simulink library "EmE_MBD_Blockset"  (R2018a)
settings: Solver=ode1  StartTime=0.0  StopTime=Inf  FixedStep=0.001  RelTol=1e-3  EnableMultiTasking=on
PostLoadFcn:
  | , if any(exist('dsrtsu_mdlpostloadfcn', 'file') == [2, 3, 6]), try dsrtsu_mdlpostloadfcn('Execute', bdroot); catch fprintf('Error in PostLoadFcn (dsrtsu_mdlpostloadfcn) for model "%s":\n %s\n', bdroot, lasterr); end, end,
undefined symbols (not defined in the file or in its folder): ENUM_TSC1_CONTROL_PURPOSE_T, gcbh, GLB_SWITCH_T
libraries: simulink x237, $bdroot x115, simulink_need_slupdate x26, MotoHawk_lib x13, simulink_extras x3
(part 8 of 11)

== system EmE_MBD_Blockset/User-Defined Functions/Snoop/CCP_ETC_SS1/Signal Data Pairing/Update Signal6/Reset Logic ==
  CurrentPID : Inport
  ResetDAQ : Inport  Port=2
  CCP_SNOOP_DAQSIZE : Constant  Value=16  OutDataTypeStr=uint8
  CCP_SNOOP_FIRSTPID : Constant  Value=64  OutDataTypeStr=uint8
  Divide : Product  Inputs=*/
  Logical Operator : Logic  Operator=OR  AllPortsSameDT=off  OutDataTypeStr=boolean
  Relational Operator : RelationalOperator  Operator===  OutDataTypeStr=boolean  RndMeth=Nearest
  Relational Operator1 : RelationalOperator  Operator===  OutDataTypeStr=boolean  RndMeth=Nearest
  Reset ALL : Constant  Value=250  OutDataTypeStr=uint8
  Subtract : Sum  Inputs=+-
  Reset : Outport
  wires:
  CCP_SNOOP_FIRSTPID/1 -> Subtract/2
  Logical Operator/1 -> Reset/1
  Relational Operator1/1 -> Logical Operator/2
  Relational Operator/1 -> Logical Operator/1
  Reset ALL/1 -> Relational Operator1/2
  ResetDAQ/1 -> Relational Operator1/1, Relational Operator/2
  Divide/1 -> Relational Operator/1  "CurrentDAQ"
  CCP_SNOOP_DAQSIZE/1 -> Divide/2
  Subtract/1 -> Divide/1
  CurrentPID/1 -> Subtract/1

== system EmE_MBD_Blockset/User-Defined Functions/Snoop/CCP_ETC_SS1/Signal Data Pairing/Update Signal7/Latch w Update ==
  f_update : Inport
  In : Inport  Port=2
  Switch : Switch  Criteria=u2 ~= 0
  Unit Delay1 : UnitDelay  SampleTime=-1
  Latched : Outport
  wires:
  Unit Delay1/1 -> Switch/3
  Switch/1 -> Unit Delay1/1, Latched/1
  In/1 -> Switch/1
  f_update/1 -> Switch/2

== system EmE_MBD_Blockset/User-Defined Functions/Snoop/CCP_ETC_SS1/Signal Data Pairing/Update Signal7/Latch w Update1 ==
  f_update : Inport
  In : Inport  Port=2
  Switch : Switch  Criteria=u2 ~= 0
  Unit Delay1 : UnitDelay  SampleTime=-1
  Latched : Outport
  wires:
  f_update/1 -> Switch/2
  In/1 -> Switch/1
  Switch/1 -> Latched/1, Unit Delay1/1
  Unit Delay1/1 -> Switch/3

== system EmE_MBD_Blockset/User-Defined Functions/Snoop/CCP_ETC_SS1/Signal Data Pairing/Update Signal7/RS Flop-Flop Rp ==
  Rp : Inport
  S : Inport  Port=2
  Logical Operator : Logic  Operator=NOT  AllPortsSameDT=off
  Logical Operator1 : Logic  AllPortsSameDT=off
  Logical Operator2 : Logic  Operator=OR  AllPortsSameDT=off
  Logical Operator3 : Logic  Operator=NOT  AllPortsSameDT=off
  Unit Delay : UnitDelay  SampleTime=-1
  Q : Outport
  !Q : Outport  Port=2
  wires:
  S/1 -> Logical Operator2/1
  Rp/1 -> Logical Operator/1
  Logical Operator3/1 -> !Q/1
  Unit Delay/1 -> Logical Operator2/2
  Logical Operator1/1 -> Unit Delay/1, Logical Operator3/1, Q/1
  Logical Operator2/1 -> Logical Operator1/2
  Logical Operator/1 -> Logical Operator1/1

== system EmE_MBD_Blockset/User-Defined Functions/Snoop/CCP_ETC_SS1/Signal Data Pairing/Update Signal7/Reset Logic ==
  CurrentPID : Inport
  ResetDAQ : Inport  Port=2
  CCP_SNOOP_DAQSIZE : Constant  Value=16  OutDataTypeStr=uint8
  CCP_SNOOP_FIRSTPID : Constant  Value=64  OutDataTypeStr=uint8
  Divide : Product  Inputs=*/
  Logical Operator : Logic  Operator=OR  AllPortsSameDT=off  OutDataTypeStr=boolean
  Relational Operator : RelationalOperator  Operator===  OutDataTypeStr=boolean  RndMeth=Nearest
  Relational Operator1 : RelationalOperator  Operator===  OutDataTypeStr=boolean  RndMeth=Nearest
  Reset ALL : Constant  Value=250  OutDataTypeStr=uint8
  Subtract : Sum  Inputs=+-
  Reset : Outport
  wires:
  CCP_SNOOP_FIRSTPID/1 -> Subtract/2
  Logical Operator/1 -> Reset/1
  Relational Operator1/1 -> Logical Operator/2
  Relational Operator/1 -> Logical Operator/1
  Reset ALL/1 -> Relational Operator1/2
  ResetDAQ/1 -> Relational Operator1/1, Relational Operator/2
  Divide/1 -> Relational Operator/1  "CurrentDAQ"
  CCP_SNOOP_DAQSIZE/1 -> Divide/2
  Subtract/1 -> Divide/1
  CurrentPID/1 -> Subtract/1

== system EmE_MBD_Blockset/User-Defined Functions/Snoop/CCP_ETC_SS1/Signal Data Pairing/Update Signal8/Latch w Update ==
  f_update : Inport
  In : Inport  Port=2
  Switch : Switch  Criteria=u2 ~= 0
  Unit Delay1 : UnitDelay  SampleTime=-1
  Latched : Outport
  wires:
  Unit Delay1/1 -> Switch/3
  Switch/1 -> Unit Delay1/1, Latched/1
  In/1 -> Switch/1
  f_update/1 -> Switch/2

== system EmE_MBD_Blockset/User-Defined Functions/Snoop/CCP_ETC_SS1/Signal Data Pairing/Update Signal8/Latch w Update1 ==
  f_update : Inport
  In : Inport  Port=2
  Switch : Switch  Criteria=u2 ~= 0
  Unit Delay1 : UnitDelay  SampleTime=-1
  Latched : Outport
  wires:
  f_update/1 -> Switch/2
  In/1 -> Switch/1
  Switch/1 -> Latched/1, Unit Delay1/1
  Unit Delay1/1 -> Switch/3

== system EmE_MBD_Blockset/User-Defined Functions/Snoop/CCP_ETC_SS1/Signal Data Pairing/Update Signal8/RS Flop-Flop Rp ==
  Rp : Inport
  S : Inport  Port=2
  Logical Operator : Logic  Operator=NOT  AllPortsSameDT=off
  Logical Operator1 : Logic  AllPortsSameDT=off
  Logical Operator2 : Logic  Operator=OR  AllPortsSameDT=off
  Logical Operator3 : Logic  Operator=NOT  AllPortsSameDT=off
  Unit Delay : UnitDelay  SampleTime=-1
  Q : Outport
  !Q : Outport  Port=2
  wires:
  S/1 -> Logical Operator2/1
  Rp/1 -> Logical Operator/1
  Logical Operator3/1 -> !Q/1
  Unit Delay/1 -> Logical Operator2/2
  Logical Operator1/1 -> Unit Delay/1, Logical Operator3/1, Q/1
  Logical Operator2/1 -> Logical Operator1/2
  Logical Operator/1 -> Logical Operator1/1

== system EmE_MBD_Blockset/User-Defined Functions/Snoop/CCP_ETC_SS1/Signal Data Pairing/Update Signal8/Reset Logic ==
  CurrentPID : Inport
  ResetDAQ : Inport  Port=2
  CCP_SNOOP_DAQSIZE : Constant  Value=16  OutDataTypeStr=uint8
  CCP_SNOOP_FIRSTPID : Constant  Value=64  OutDataTypeStr=uint8
  Divide : Product  Inputs=*/
  Logical Operator : Logic  Operator=OR  AllPortsSameDT=off  OutDataTypeStr=boolean
  Relational Operator : RelationalOperator  Operator===  OutDataTypeStr=boolean  RndMeth=Nearest
  Relational Operator1 : RelationalOperator  Operator===  OutDataTypeStr=boolean  RndMeth=Nearest
  Reset ALL : Constant  Value=250  OutDataTypeStr=uint8
  Subtract : Sum  Inputs=+-
  Reset : Outport
  wires:
  CCP_SNOOP_FIRSTPID/1 -> Subtract/2
  Logical Operator/1 -> Reset/1
  Relational Operator1/1 -> Logical Operator/2
  Relational Operator/1 -> Logical Operator/1
  Reset ALL/1 -> Relational Operator1/2
  ResetDAQ/1 -> Relational Operator1/1, Relational Operator/2
  Divide/1 -> Relational Operator/1  "CurrentDAQ"
  CCP_SNOOP_DAQSIZE/1 -> Divide/2
  Subtract/1 -> Divide/1
  CurrentPID/1 -> Subtract/1

== system EmE_MBD_Blockset/User-Defined Functions/Snoop/CCP_ETC_SS1/Signal Data Pairing/Update Signal9/Latch w Update ==
  f_update : Inport
  In : Inport  Port=2
  Switch : Switch  Criteria=u2 ~= 0
  Unit Delay1 : UnitDelay  SampleTime=-1
  Latched : Outport
  wires:
  Unit Delay1/1 -> Switch/3
  Switch/1 -> Unit Delay1/1, Latched/1
  In/1 -> Switch/1
  f_update/1 -> Switch/2

== system EmE_MBD_Blockset/User-Defined Functions/Snoop/CCP_ETC_SS1/Signal Data Pairing/Update Signal9/Latch w Update1 ==
  f_update : Inport
  In : Inport  Port=2
  Switch : Switch  Criteria=u2 ~= 0
  Unit Delay1 : UnitDelay  SampleTime=-1
  Latched : Outport
  wires:
  f_update/1 -> Switch/2
  In/1 -> Switch/1
  Switch/1 -> Latched/1, Unit Delay1/1
  Unit Delay1/1 -> Switch/3

== system EmE_MBD_Blockset/User-Defined Functions/Snoop/CCP_ETC_SS1/Signal Data Pairing/Update Signal9/RS Flop-Flop Rp ==
  Rp : Inport
  S : Inport  Port=2
  Logical Operator : Logic  Operator=NOT  AllPortsSameDT=off
  Logical Operator1 : Logic  AllPortsSameDT=off
  Logical Operator2 : Logic  Operator=OR  AllPortsSameDT=off
  Logical Operator3 : Logic  Operator=NOT  AllPortsSameDT=off
  Unit Delay : UnitDelay  SampleTime=-1
  Q : Outport
  !Q : Outport  Port=2
  wires:
  S/1 -> Logical Operator2/1
  Rp/1 -> Logical Operator/1
  Logical Operator3/1 -> !Q/1
  Unit Delay/1 -> Logical Operator2/2
  Logical Operator1/1 -> Unit Delay/1, Logical Operator3/1, Q/1
  Logical Operator2/1 -> Logical Operator1/2
  Logical Operator/1 -> Logical Operator1/1

== system EmE_MBD_Blockset/User-Defined Functions/Snoop/CCP_ETC_SS1/Signal Data Pairing/Update Signal9/Reset Logic ==
  CurrentPID : Inport
  ResetDAQ : Inport  Port=2
  CCP_SNOOP_DAQSIZE : Constant  Value=16  OutDataTypeStr=uint8
  CCP_SNOOP_FIRSTPID : Constant  Value=64  OutDataTypeStr=uint8
  Divide : Product  Inputs=*/
  Logical Operator : Logic  Operator=OR  AllPortsSameDT=off  OutDataTypeStr=boolean
  Relational Operator : RelationalOperator  Operator===  OutDataTypeStr=boolean  RndMeth=Nearest
  Relational Operator1 : RelationalOperator  Operator===  OutDataTypeStr=boolean  RndMeth=Nearest
  Reset ALL : Constant  Value=250  OutDataTypeStr=uint8
  Subtract : Sum  Inputs=+-
  Reset : Outport
  wires:
  CCP_SNOOP_FIRSTPID/1 -> Subtract/2
  Logical Operator/1 -> Reset/1
  Relational Operator1/1 -> Logical Operator/2
  Relational Operator/1 -> Logical Operator/1
  Reset ALL/1 -> Relational Operator1/2
  ResetDAQ/1 -> Relational Operator1/1, Relational Operator/2
  Divide/1 -> Relational Operator/1  "CurrentDAQ"
  CCP_SNOOP_DAQSIZE/1 -> Divide/2
  Subtract/1 -> Divide/1
  CurrentPID/1 -> Subtract/1

== system EmE_MBD_Blockset/User-Defined Functions/Snoop/CCP_ETC_SS2/CCP_Parameter_Decode/Decode_Signal1/Isolate Data ==
  Offset : Inport
  Data : Inport  Port=2
  Type : Inport  Port=3
  1Byte : Subsystem
  2Bytes : Subsystem
  4Bytes : Subsystem
  Constant1 : Constant
  Constant2 : Constant  Value=2
  Data Type Conversion{,1..7} (8 alike) : DataTypeConversion  OutDataTypeStr=uint8
  Demux : Demux  Outputs=8
  Mux : Mux  Inputs=7
  Relational Operator : RelationalOperator  Operator===  OutDataTypeStr=boolean  RndMeth=Nearest
  Relational Operator1 : RelationalOperator  Operator===  OutDataTypeStr=boolean  RndMeth=Nearest
  Size : Subsystem
  Switch1 : Switch  Criteria=u2 ~= 0
  Switch2 : Switch  Criteria=u2 ~= 0
  Terminator : Terminator
  Raw32 : Outport
  wires:
  Data Type Conversion/1 -> Terminator/1  "PID"
  Demux/8 -> Data Type Conversion7/1
  Demux/7 -> Data Type Conversion6/1
  Demux/6 -> Data Type Conversion5/1
  Demux/5 -> Data Type Conversion4/1
  Demux/4 -> Data Type Conversion3/1
  Demux/3 -> Data Type Conversion2/1
  Demux/2 -> Data Type Conversion1/1
  Demux/1 -> Data Type Conversion/1
  Data/1 -> Demux/1
  Offset/1 -> [offset]
  Data Type Conversion1/1 -> Mux/1  "0"
  Data Type Conversion2/1 -> Mux/2  "1"
  Data Type Conversion3/1 -> Mux/3  "2"
  Data Type Conversion4/1 -> Mux/4  "3"
  Data Type Conversion5/1 -> Mux/5  "4"
  Data Type Conversion6/1 -> Mux/6  "5"
  Data Type Conversion7/1 -> Mux/7  "6"
  Type/1 -> Size/1(Type)
  Size/1(Byte_Count) -> Relational Operator/1, Relational Operator1/1
  Switch1/1 -> Switch2/3
  Constant1/1 -> Relational Operator/2
  Constant2/1 -> Relational Operator1/2
  Relational Operator/1 -> Switch2/2
  Relational Operator1/1 -> Switch1/2
  1Byte/1(Y) -> Switch2/1
  [offset] -> 1Byte/2(Idx)
  [data] -> 1Byte/1(U)
  2Bytes/1(Y) -> Switch1/1
  Mux/1 -> 2Bytes/1(U), [data], 4Bytes/1(U)
  [offset] -> 2Bytes/2(Idx1)
  [offset] -> 4Bytes/2(Idx)
  Switch2/1 -> Raw32/1
  4Bytes/1(Y) -> Switch1/3

== system EmE_MBD_Blockset/User-Defined Functions/Snoop/CCP_ETC_SS2/CCP_Parameter_Decode/Decode_Signal1/Signal Decode ==
  Raw32 : Inport
  Type : Inport  Port=2
  Coversion : Inport  Port=3
  Bitwise Operator : simulink/Logic and Bit Operations/Bitwise Operator  logicop=AND  UseBitMask=on  BitMask=bin2dec('00000001')  BitMaskRealWorld=Stored Integer
  FLOAT32 : Subsystem
  Integer_Data : Subsystem
  Switch1 : Switch  Criteria=u2 ~= 0
  Unit_Convert : Subsystem
  Out1 : Outport
  wires:
  Unit_Convert/1(Scaled) -> Switch1/1
  Integer_Data/1(Raw) -> Unit_Convert/1(Raw)
  Switch1/1 -> Out1/1
  Bitwise Operator/1 -> Switch1/2
  Raw32/1 -> FLOAT32/1(Raw32), Integer_Data/2(Raw32)
  Type/1 -> Bitwise Operator/1, Integer_Data/1(Type)
  FLOAT32/1(Raw) -> Switch1/3
  Coversion/1 -> Unit_Convert/2(Conversion)

== system EmE_MBD_Blockset/User-Defined Functions/Snoop/CCP_ETC_SS2/CCP_Parameter_Decode/Decode_Signal10/Isolate Data ==
  Offset : Inport
  Data : Inport  Port=2
  Type : Inport  Port=3
  1Byte : Subsystem
  2Bytes : Subsystem
  4Bytes : Subsystem
  Constant1 : Constant
  Constant2 : Constant  Value=2
  Data Type Conversion{,1..7} (8 alike) : DataTypeConversion  OutDataTypeStr=uint8
  Demux : Demux  Outputs=8
  Mux : Mux  Inputs=7
  Relational Operator : RelationalOperator  Operator===  OutDataTypeStr=boolean  RndMeth=Nearest
  Relational Operator1 : RelationalOperator  Operator===  OutDataTypeStr=boolean  RndMeth=Nearest
  Size : Subsystem
  Switch1 : Switch  Criteria=u2 ~= 0
  Switch2 : Switch  Criteria=u2 ~= 0
  Terminator : Terminator
  Raw32 : Outport
  wires:
  4Bytes/1(Y) -> Switch1/3
  Switch2/1 -> Raw32/1
  [offset] -> 4Bytes/2(Idx)
  [offset] -> 2Bytes/2(Idx1)
  Mux/1 -> 4Bytes/1(U), [data], 2Bytes/1(U)
  2Bytes/1(Y) -> Switch1/1
  [data] -> 1Byte/1(U)
  [offset] -> 1Byte/2(Idx)
  1Byte/1(Y) -> Switch2/1
  Relational Operator1/1 -> Switch1/2
  Relational Operator/1 -> Switch2/2
  Constant2/1 -> Relational Operator1/2
  Constant1/1 -> Relational Operator/2
  Switch1/1 -> Switch2/3
  Size/1(Byte_Count) -> Relational Operator1/1, Relational Operator/1
  Type/1 -> Size/1(Type)
  Data Type Conversion7/1 -> Mux/7  "6"
  Data Type Conversion6/1 -> Mux/6  "5"
  Data Type Conversion5/1 -> Mux/5  "4"
  Data Type Conversion4/1 -> Mux/4  "3"
  Data Type Conversion3/1 -> Mux/3  "2"
  Data Type Conversion2/1 -> Mux/2  "1"
  Data Type Conversion1/1 -> Mux/1  "0"
  Offset/1 -> [offset]
  Data/1 -> Demux/1
  Demux/1 -> Data Type Conversion/1
  Demux/2 -> Data Type Conversion1/1
  Demux/3 -> Data Type Conversion2/1
  Demux/4 -> Data Type Conversion3/1
  Demux/5 -> Data Type Conversion4/1
  Demux/6 -> Data Type Conversion5/1
  Demux/7 -> Data Type Conversion6/1
  Demux/8 -> Data Type Conversion7/1
  Data Type Conversion/1 -> Terminator/1  "PID"

== system EmE_MBD_Blockset/User-Defined Functions/Snoop/CCP_ETC_SS2/CCP_Parameter_Decode/Decode_Signal10/Signal Decode ==
  Raw32 : Inport
  Type : Inport  Port=2
  Coversion : Inport  Port=3
  Bitwise Operator : simulink/Logic and Bit Operations/Bitwise Operator  logicop=AND  UseBitMask=on  BitMask=bin2dec('00000001')  BitMaskRealWorld=Stored Integer
  FLOAT32 : Subsystem
  Integer_Data : Subsystem
  Switch1 : Switch  Criteria=u2 ~= 0
  Unit_Convert : Subsystem
  Out1 : Outport
  wires:
  Coversion/1 -> Unit_Convert/2(Conversion)
  FLOAT32/1(Raw) -> Switch1/3
  Type/1 -> Integer_Data/1(Type), Bitwise Operator/1
  Raw32/1 -> Integer_Data/2(Raw32), FLOAT32/1(Raw32)
  Bitwise Operator/1 -> Switch1/2
  Switch1/1 -> Out1/1
  Integer_Data/1(Raw) -> Unit_Convert/1(Raw)
  Unit_Convert/1(Scaled) -> Switch1/1

== system EmE_MBD_Blockset/User-Defined Functions/Snoop/CCP_ETC_SS2/CCP_Parameter_Decode/Decode_Signal11/Isolate Data ==
  Offset : Inport
  Data : Inport  Port=2
  Type : Inport  Port=3
  1Byte : Subsystem
  2Bytes : Subsystem
  4Bytes : Subsystem
  Constant1 : Constant
  Constant2 : Constant  Value=2
  Data Type Conversion{,1..7} (8 alike) : DataTypeConversion  OutDataTypeStr=uint8
  Demux : Demux  Outputs=8
  Mux : Mux  Inputs=7
  Relational Operator : RelationalOperator  Operator===  OutDataTypeStr=boolean  RndMeth=Nearest
  Relational Operator1 : RelationalOperator  Operator===  OutDataTypeStr=boolean  RndMeth=Nearest
  Size : Subsystem
  Switch1 : Switch  Criteria=u2 ~= 0
  Switch2 : Switch  Criteria=u2 ~= 0
  Terminator : Terminator
  Raw32 : Outport
  wires:
  Data Type Conversion/1 -> Terminator/1  "PID"
  Demux/8 -> Data Type Conversion7/1
  Demux/7 -> Data Type Conversion6/1
  Demux/6 -> Data Type Conversion5/1
  Demux/5 -> Data Type Conversion4/1
  Demux/4 -> Data Type Conversion3/1
  Demux/3 -> Data Type Conversion2/1
  Demux/2 -> Data Type Conversion1/1
  Demux/1 -> Data Type Conversion/1
  Data/1 -> Demux/1
  Offset/1 -> [offset]
  Data Type Conversion1/1 -> Mux/1  "0"
  Data Type Conversion2/1 -> Mux/2  "1"
  Data Type Conversion3/1 -> Mux/3  "2"
  Data Type Conversion4/1 -> Mux/4  "3"
  Data Type Conversion5/1 -> Mux/5  "4"
  Data Type Conversion6/1 -> Mux/6  "5"
  Data Type Conversion7/1 -> Mux/7  "6"
  Type/1 -> Size/1(Type)
  Size/1(Byte_Count) -> Relational Operator/1, Relational Operator1/1
  Switch1/1 -> Switch2/3
  Constant1/1 -> Relational Operator/2
  Constant2/1 -> Relational Operator1/2
  Relational Operator/1 -> Switch2/2
  Relational Operator1/1 -> Switch1/2
  1Byte/1(Y) -> Switch2/1
  [offset] -> 1Byte/2(Idx)
  [data] -> 1Byte/1(U)
  2Bytes/1(Y) -> Switch1/1
  Mux/1 -> 2Bytes/1(U), [data], 4Bytes/1(U)
  [offset] -> 2Bytes/2(Idx1)
  [offset] -> 4Bytes/2(Idx)
  Switch2/1 -> Raw32/1
  4Bytes/1(Y) -> Switch1/3

== system EmE_MBD_Blockset/User-Defined Functions/Snoop/CCP_ETC_SS2/CCP_Parameter_Decode/Decode_Signal11/Signal Decode ==
  Raw32 : Inport
  Type : Inport  Port=2
  Coversion : Inport  Port=3
  Bitwise Operator : simulink/Logic and Bit Operations/Bitwise Operator  logicop=AND  UseBitMask=on  BitMask=bin2dec('00000001')  BitMaskRealWorld=Stored Integer
  FLOAT32 : Subsystem
  Integer_Data : Subsystem
  Switch1 : Switch  Criteria=u2 ~= 0
  Unit_Convert : Subsystem
  Out1 : Outport
  wires:
  Unit_Convert/1(Scaled) -> Switch1/1
  Integer_Data/1(Raw) -> Unit_Convert/1(Raw)
  Switch1/1 -> Out1/1
  Bitwise Operator/1 -> Switch1/2
  Raw32/1 -> FLOAT32/1(Raw32), Integer_Data/2(Raw32)
  Type/1 -> Bitwise Operator/1, Integer_Data/1(Type)
  FLOAT32/1(Raw) -> Switch1/3
  Coversion/1 -> Unit_Convert/2(Conversion)

== system EmE_MBD_Blockset/User-Defined Functions/Snoop/CCP_ETC_SS2/CCP_Parameter_Decode/Decode_Signal12/Isolate Data ==
  Offset : Inport
  Data : Inport  Port=2
  Type : Inport  Port=3
  1Byte : Subsystem
  2Bytes : Subsystem
  4Bytes : Subsystem
  Constant1 : Constant
  Constant2 : Constant  Value=2
  Data Type Conversion{,1..7} (8 alike) : DataTypeConversion  OutDataTypeStr=uint8
  Demux : Demux  Outputs=8
  Mux : Mux  Inputs=7
  Relational Operator : RelationalOperator  Operator===  OutDataTypeStr=boolean  RndMeth=Nearest
  Relational Operator1 : RelationalOperator  Operator===  OutDataTypeStr=boolean  RndMeth=Nearest
  Size : Subsystem
  Switch1 : Switch  Criteria=u2 ~= 0
  Switch2 : Switch  Criteria=u2 ~= 0
  Terminator : Terminator
  Raw32 : Outport
  wires:
  4Bytes/1(Y) -> Switch1/3
  Switch2/1 -> Raw32/1
  [offset] -> 4Bytes/2(Idx)
  [offset] -> 2Bytes/2(Idx1)
  Mux/1 -> 4Bytes/1(U), [data], 2Bytes/1(U)
  2Bytes/1(Y) -> Switch1/1
  [data] -> 1Byte/1(U)
  [offset] -> 1Byte/2(Idx)
  1Byte/1(Y) -> Switch2/1
  Relational Operator1/1 -> Switch1/2
  Relational Operator/1 -> Switch2/2
  Constant2/1 -> Relational Operator1/2
  Constant1/1 -> Relational Operator/2
  Switch1/1 -> Switch2/3
  Size/1(Byte_Count) -> Relational Operator1/1, Relational Operator/1
  Type/1 -> Size/1(Type)
  Data Type Conversion7/1 -> Mux/7  "6"
  Data Type Conversion6/1 -> Mux/6  "5"
  Data Type Conversion5/1 -> Mux/5  "4"
  Data Type Conversion4/1 -> Mux/4  "3"
  Data Type Conversion3/1 -> Mux/3  "2"
  Data Type Conversion2/1 -> Mux/2  "1"
  Data Type Conversion1/1 -> Mux/1  "0"
  Offset/1 -> [offset]
  Data/1 -> Demux/1
  Demux/1 -> Data Type Conversion/1
  Demux/2 -> Data Type Conversion1/1
  Demux/3 -> Data Type Conversion2/1
  Demux/4 -> Data Type Conversion3/1
  Demux/5 -> Data Type Conversion4/1
  Demux/6 -> Data Type Conversion5/1
  Demux/7 -> Data Type Conversion6/1
  Demux/8 -> Data Type Conversion7/1
  Data Type Conversion/1 -> Terminator/1  "PID"

== system EmE_MBD_Blockset/User-Defined Functions/Snoop/CCP_ETC_SS2/CCP_Parameter_Decode/Decode_Signal12/Signal Decode ==
  Raw32 : Inport
  Type : Inport  Port=2
  Coversion : Inport  Port=3
  Bitwise Operator : simulink/Logic and Bit Operations/Bitwise Operator  logicop=AND  UseBitMask=on  BitMask=bin2dec('00000001')  BitMaskRealWorld=Stored Integer
  FLOAT32 : Subsystem
  Integer_Data : Subsystem
  Switch1 : Switch  Criteria=u2 ~= 0
  Unit_Convert : Subsystem
  Out1 : Outport
  wires:
  Coversion/1 -> Unit_Convert/2(Conversion)
  FLOAT32/1(Raw) -> Switch1/3
  Type/1 -> Integer_Data/1(Type), Bitwise Operator/1
  Raw32/1 -> Integer_Data/2(Raw32), FLOAT32/1(Raw32)
  Bitwise Operator/1 -> Switch1/2
  Switch1/1 -> Out1/1
  Integer_Data/1(Raw) -> Unit_Convert/1(Raw)
  Unit_Convert/1(Scaled) -> Switch1/1

== system EmE_MBD_Blockset/User-Defined Functions/Snoop/CCP_ETC_SS2/CCP_Parameter_Decode/Decode_Signal2/Isolate Data ==
  Offset : Inport
  Data : Inport  Port=2
  Type : Inport  Port=3
  1Byte : Subsystem
  2Bytes : Subsystem
  4Bytes : Subsystem
  Constant1 : Constant
  Constant2 : Constant  Value=2
  Data Type Conversion{,1..7} (8 alike) : DataTypeConversion  OutDataTypeStr=uint8
  Demux : Demux  Outputs=8
  Mux : Mux  Inputs=7
  Relational Operator : RelationalOperator  Operator===  OutDataTypeStr=boolean  RndMeth=Nearest
  Relational Operator1 : RelationalOperator  Operator===  OutDataTypeStr=boolean  RndMeth=Nearest
  Size : Subsystem
  Switch1 : Switch  Criteria=u2 ~= 0
  Switch2 : Switch  Criteria=u2 ~= 0
  Terminator : Terminator
  Raw32 : Outport
  wires:
  4Bytes/1(Y) -> Switch1/3
  Switch2/1 -> Raw32/1
  [offset] -> 4Bytes/2(Idx)
  [offset] -> 2Bytes/2(Idx1)
  Mux/1 -> 4Bytes/1(U), [data], 2Bytes/1(U)
  2Bytes/1(Y) -> Switch1/1
  [data] -> 1Byte/1(U)
  [offset] -> 1Byte/2(Idx)
  1Byte/1(Y) -> Switch2/1
  Relational Operator1/1 -> Switch1/2
  Relational Operator/1 -> Switch2/2
  Constant2/1 -> Relational Operator1/2
  Constant1/1 -> Relational Operator/2
  Switch1/1 -> Switch2/3
  Size/1(Byte_Count) -> Relational Operator1/1, Relational Operator/1
  Type/1 -> Size/1(Type)
  Data Type Conversion7/1 -> Mux/7  "6"
  Data Type Conversion6/1 -> Mux/6  "5"
  Data Type Conversion5/1 -> Mux/5  "4"
  Data Type Conversion4/1 -> Mux/4  "3"
  Data Type Conversion3/1 -> Mux/3  "2"
  Data Type Conversion2/1 -> Mux/2  "1"
  Data Type Conversion1/1 -> Mux/1  "0"
  Offset/1 -> [offset]
  Data/1 -> Demux/1
  Demux/1 -> Data Type Conversion/1
  Demux/2 -> Data Type Conversion1/1
  Demux/3 -> Data Type Conversion2/1
  Demux/4 -> Data Type Conversion3/1
  Demux/5 -> Data Type Conversion4/1
  Demux/6 -> Data Type Conversion5/1
  Demux/7 -> Data Type Conversion6/1
  Demux/8 -> Data Type Conversion7/1
  Data Type Conversion/1 -> Terminator/1  "PID"

== system EmE_MBD_Blockset/User-Defined Functions/Snoop/CCP_ETC_SS2/CCP_Parameter_Decode/Decode_Signal2/Signal Decode ==
  Raw32 : Inport
  Type : Inport  Port=2
  Coversion : Inport  Port=3
  Bitwise Operator : simulink/Logic and Bit Operations/Bitwise Operator  logicop=AND  UseBitMask=on  BitMask=bin2dec('00000001')  BitMaskRealWorld=Stored Integer
  FLOAT32 : Subsystem
  Integer_Data : Subsystem
  Switch1 : Switch  Criteria=u2 ~= 0
  Unit_Convert : Subsystem
  Out1 : Outport
  wires:
  Coversion/1 -> Unit_Convert/2(Conversion)
  FLOAT32/1(Raw) -> Switch1/3
  Type/1 -> Integer_Data/1(Type), Bitwise Operator/1
  Raw32/1 -> Integer_Data/2(Raw32), FLOAT32/1(Raw32)
  Bitwise Operator/1 -> Switch1/2
  Switch1/1 -> Out1/1
  Integer_Data/1(Raw) -> Unit_Convert/1(Raw)
  Unit_Convert/1(Scaled) -> Switch1/1

== system EmE_MBD_Blockset/User-Defined Functions/Snoop/CCP_ETC_SS2/CCP_Parameter_Decode/Decode_Signal3/Isolate Data ==
  Offset : Inport
  Data : Inport  Port=2
  Type : Inport  Port=3
  1Byte : Subsystem
  2Bytes : Subsystem
  4Bytes : Subsystem
  Constant1 : Constant
  Constant2 : Constant  Value=2
  Data Type Conversion{,1..7} (8 alike) : DataTypeConversion  OutDataTypeStr=uint8
  Demux : Demux  Outputs=8
  Mux : Mux  Inputs=7
  Relational Operator : RelationalOperator  Operator===  OutDataTypeStr=boolean  RndMeth=Nearest
  Relational Operator1 : RelationalOperator  Operator===  OutDataTypeStr=boolean  RndMeth=Nearest
  Size : Subsystem
  Switch1 : Switch  Criteria=u2 ~= 0
  Switch2 : Switch  Criteria=u2 ~= 0
  Terminator : Terminator
  Raw32 : Outport
  wires:
  Data Type Conversion/1 -> Terminator/1  "PID"
  Demux/8 -> Data Type Conversion7/1
  Demux/7 -> Data Type Conversion6/1
  Demux/6 -> Data Type Conversion5/1
  Demux/5 -> Data Type Conversion4/1
  Demux/4 -> Data Type Conversion3/1
  Demux/3 -> Data Type Conversion2/1
  Demux/2 -> Data Type Conversion1/1
  Demux/1 -> Data Type Conversion/1
  Data/1 -> Demux/1
  Offset/1 -> [offset]
  Data Type Conversion1/1 -> Mux/1  "0"
  Data Type Conversion2/1 -> Mux/2  "1"
  Data Type Conversion3/1 -> Mux/3  "2"
  Data Type Conversion4/1 -> Mux/4  "3"
  Data Type Conversion5/1 -> Mux/5  "4"
  Data Type Conversion6/1 -> Mux/6  "5"
  Data Type Conversion7/1 -> Mux/7  "6"
  Type/1 -> Size/1(Type)
  Size/1(Byte_Count) -> Relational Operator/1, Relational Operator1/1
  Switch1/1 -> Switch2/3
  Constant1/1 -> Relational Operator/2
  Constant2/1 -> Relational Operator1/2
  Relational Operator/1 -> Switch2/2
  Relational Operator1/1 -> Switch1/2
  1Byte/1(Y) -> Switch2/1
  [offset] -> 1Byte/2(Idx)
  [data] -> 1Byte/1(U)
  2Bytes/1(Y) -> Switch1/1
  Mux/1 -> 2Bytes/1(U), [data], 4Bytes/1(U)
  [offset] -> 2Bytes/2(Idx1)
  [offset] -> 4Bytes/2(Idx)
  Switch2/1 -> Raw32/1
  4Bytes/1(Y) -> Switch1/3

== system EmE_MBD_Blockset/User-Defined Functions/Snoop/CCP_ETC_SS2/CCP_Parameter_Decode/Decode_Signal3/Signal Decode ==
  Raw32 : Inport
  Type : Inport  Port=2
  Coversion : Inport  Port=3
  Bitwise Operator : simulink/Logic and Bit Operations/Bitwise Operator  logicop=AND  UseBitMask=on  BitMask=bin2dec('00000001')  BitMaskRealWorld=Stored Integer
  FLOAT32 : Subsystem
  Integer_Data : Subsystem
  Switch1 : Switch  Criteria=u2 ~= 0
  Unit_Convert : Subsystem
  Out1 : Outport
  wires:
  Unit_Convert/1(Scaled) -> Switch1/1
  Integer_Data/1(Raw) -> Unit_Convert/1(Raw)
  Switch1/1 -> Out1/1
  Bitwise Operator/1 -> Switch1/2
  Raw32/1 -> FLOAT32/1(Raw32), Integer_Data/2(Raw32)
  Type/1 -> Bitwise Operator/1, Integer_Data/1(Type)
  FLOAT32/1(Raw) -> Switch1/3
  Coversion/1 -> Unit_Convert/2(Conversion)

== system EmE_MBD_Blockset/User-Defined Functions/Snoop/CCP_ETC_SS2/CCP_Parameter_Decode/Decode_Signal4/Isolate Data ==
  Offset : Inport
  Data : Inport  Port=2
  Type : Inport  Port=3
  1Byte : Subsystem
  2Bytes : Subsystem
  4Bytes : Subsystem
  Constant1 : Constant
  Constant2 : Constant  Value=2
  Data Type Conversion{,1..7} (8 alike) : DataTypeConversion  OutDataTypeStr=uint8
  Demux : Demux  Outputs=8
  Mux : Mux  Inputs=7
  Relational Operator : RelationalOperator  Operator===  OutDataTypeStr=boolean  RndMeth=Nearest
  Relational Operator1 : RelationalOperator  Operator===  OutDataTypeStr=boolean  RndMeth=Nearest
  Size : Subsystem
  Switch1 : Switch  Criteria=u2 ~= 0
  Switch2 : Switch  Criteria=u2 ~= 0
  Terminator : Terminator
  Raw32 : Outport
  wires:
  4Bytes/1(Y) -> Switch1/3
  Switch2/1 -> Raw32/1
  [offset] -> 4Bytes/2(Idx)
  [offset] -> 2Bytes/2(Idx1)
  Mux/1 -> 4Bytes/1(U), [data], 2Bytes/1(U)
  2Bytes/1(Y) -> Switch1/1
  [data] -> 1Byte/1(U)
  [offset] -> 1Byte/2(Idx)
  1Byte/1(Y) -> Switch2/1
  Relational Operator1/1 -> Switch1/2
  Relational Operator/1 -> Switch2/2
  Constant2/1 -> Relational Operator1/2
  Constant1/1 -> Relational Operator/2
  Switch1/1 -> Switch2/3
  Size/1(Byte_Count) -> Relational Operator1/1, Relational Operator/1
  Type/1 -> Size/1(Type)
  Data Type Conversion7/1 -> Mux/7  "6"
  Data Type Conversion6/1 -> Mux/6  "5"
  Data Type Conversion5/1 -> Mux/5  "4"
  Data Type Conversion4/1 -> Mux/4  "3"
  Data Type Conversion3/1 -> Mux/3  "2"
  Data Type Conversion2/1 -> Mux/2  "1"
  Data Type Conversion1/1 -> Mux/1  "0"
  Offset/1 -> [offset]
  Data/1 -> Demux/1
  Demux/1 -> Data Type Conversion/1
  Demux/2 -> Data Type Conversion1/1
  Demux/3 -> Data Type Conversion2/1
  Demux/4 -> Data Type Conversion3/1
  Demux/5 -> Data Type Conversion4/1
  Demux/6 -> Data Type Conversion5/1
  Demux/7 -> Data Type Conversion6/1
  Demux/8 -> Data Type Conversion7/1
  Data Type Conversion/1 -> Terminator/1  "PID"

== system EmE_MBD_Blockset/User-Defined Functions/Snoop/CCP_ETC_SS2/CCP_Parameter_Decode/Decode_Signal4/Signal Decode ==
  Raw32 : Inport
  Type : Inport  Port=2
  Coversion : Inport  Port=3
  Bitwise Operator : simulink/Logic and Bit Operations/Bitwise Operator  logicop=AND  UseBitMask=on  BitMask=bin2dec('00000001')  BitMaskRealWorld=Stored Integer
  FLOAT32 : Subsystem
  Integer_Data : Subsystem
  Switch1 : Switch  Criteria=u2 ~= 0
  Unit_Convert : Subsystem
  Out1 : Outport
  wires:
  Coversion/1 -> Unit_Convert/2(Conversion)
  FLOAT32/1(Raw) -> Switch1/3
  Type/1 -> Integer_Data/1(Type), Bitwise Operator/1
  Raw32/1 -> Integer_Data/2(Raw32), FLOAT32/1(Raw32)
  Bitwise Operator/1 -> Switch1/2
  Switch1/1 -> Out1/1
  Integer_Data/1(Raw) -> Unit_Convert/1(Raw)
  Unit_Convert/1(Scaled) -> Switch1/1

== system EmE_MBD_Blockset/User-Defined Functions/Snoop/CCP_ETC_SS2/CCP_Parameter_Decode/Decode_Signal5/Isolate Data ==
  Offset : Inport
  Data : Inport  Port=2
  Type : Inport  Port=3
  1Byte : Subsystem
  2Bytes : Subsystem
  4Bytes : Subsystem
  Constant1 : Constant
  Constant2 : Constant  Value=2
  Data Type Conversion{,1..7} (8 alike) : DataTypeConversion  OutDataTypeStr=uint8
  Demux : Demux  Outputs=8
  Mux : Mux  Inputs=7
  Relational Operator : RelationalOperator  Operator===  OutDataTypeStr=boolean  RndMeth=Nearest
  Relational Operator1 : RelationalOperator  Operator===  OutDataTypeStr=boolean  RndMeth=Nearest
  Size : Subsystem
  Switch1 : Switch  Criteria=u2 ~= 0
  Switch2 : Switch  Criteria=u2 ~= 0
  Terminator : Terminator
  Raw32 : Outport
  wires:
  Data Type Conversion/1 -> Terminator/1  "PID"
  Demux/8 -> Data Type Conversion7/1
  Demux/7 -> Data Type Conversion6/1
  Demux/6 -> Data Type Conversion5/1
  Demux/5 -> Data Type Conversion4/1
  Demux/4 -> Data Type Conversion3/1
  Demux/3 -> Data Type Conversion2/1
  Demux/2 -> Data Type Conversion1/1
  Demux/1 -> Data Type Conversion/1
  Data/1 -> Demux/1
  Offset/1 -> [offset]
  Data Type Conversion1/1 -> Mux/1  "0"
  Data Type Conversion2/1 -> Mux/2  "1"
  Data Type Conversion3/1 -> Mux/3  "2"
  Data Type Conversion4/1 -> Mux/4  "3"
  Data Type Conversion5/1 -> Mux/5  "4"
  Data Type Conversion6/1 -> Mux/6  "5"
  Data Type Conversion7/1 -> Mux/7  "6"
  Type/1 -> Size/1(Type)
  Size/1(Byte_Count) -> Relational Operator/1, Relational Operator1/1
  Switch1/1 -> Switch2/3
  Constant1/1 -> Relational Operator/2
  Constant2/1 -> Relational Operator1/2
  Relational Operator/1 -> Switch2/2
  Relational Operator1/1 -> Switch1/2
  1Byte/1(Y) -> Switch2/1
  [offset] -> 1Byte/2(Idx)
  [data] -> 1Byte/1(U)
  2Bytes/1(Y) -> Switch1/1
  Mux/1 -> 2Bytes/1(U), [data], 4Bytes/1(U)
  [offset] -> 2Bytes/2(Idx1)
  [offset] -> 4Bytes/2(Idx)
  Switch2/1 -> Raw32/1
  4Bytes/1(Y) -> Switch1/3

== system EmE_MBD_Blockset/User-Defined Functions/Snoop/CCP_ETC_SS2/CCP_Parameter_Decode/Decode_Signal5/Signal Decode ==
  Raw32 : Inport
  Type : Inport  Port=2
  Coversion : Inport  Port=3
  Bitwise Operator : simulink/Logic and Bit Operations/Bitwise Operator  logicop=AND  UseBitMask=on  BitMask=bin2dec('00000001')  BitMaskRealWorld=Stored Integer
  FLOAT32 : Subsystem
  Integer_Data : Subsystem
  Switch1 : Switch  Criteria=u2 ~= 0
  Unit_Convert : Subsystem
  Out1 : Outport
  wires:
  Unit_Convert/1(Scaled) -> Switch1/1
  Integer_Data/1(Raw) -> Unit_Convert/1(Raw)
  Switch1/1 -> Out1/1
  Bitwise Operator/1 -> Switch1/2
  Raw32/1 -> FLOAT32/1(Raw32), Integer_Data/2(Raw32)
  Type/1 -> Bitwise Operator/1, Integer_Data/1(Type)
  FLOAT32/1(Raw) -> Switch1/3
  Coversion/1 -> Unit_Convert/2(Conversion)

== system EmE_MBD_Blockset/User-Defined Functions/Snoop/CCP_ETC_SS2/CCP_Parameter_Decode/Decode_Signal6/Isolate Data ==
  Offset : Inport
  Data : Inport  Port=2
  Type : Inport  Port=3
  1Byte : Subsystem
  2Bytes : Subsystem
  4Bytes : Subsystem
  Constant1 : Constant
  Constant2 : Constant  Value=2
  Data Type Conversion{,1..7} (8 alike) : DataTypeConversion  OutDataTypeStr=uint8
  Demux : Demux  Outputs=8
  Mux : Mux  Inputs=7
  Relational Operator : RelationalOperator  Operator===  OutDataTypeStr=boolean  RndMeth=Nearest
  Relational Operator1 : RelationalOperator  Operator===  OutDataTypeStr=boolean  RndMeth=Nearest
  Size : Subsystem
  Switch1 : Switch  Criteria=u2 ~= 0
  Switch2 : Switch  Criteria=u2 ~= 0
  Terminator : Terminator
  Raw32 : Outport
  wires:
  4Bytes/1(Y) -> Switch1/3
  Switch2/1 -> Raw32/1
  [offset] -> 4Bytes/2(Idx)
  [offset] -> 2Bytes/2(Idx1)
  Mux/1 -> 4Bytes/1(U), [data], 2Bytes/1(U)
  2Bytes/1(Y) -> Switch1/1
  [data] -> 1Byte/1(U)
  [offset] -> 1Byte/2(Idx)
  1Byte/1(Y) -> Switch2/1
  Relational Operator1/1 -> Switch1/2
  Relational Operator/1 -> Switch2/2
  Constant2/1 -> Relational Operator1/2
  Constant1/1 -> Relational Operator/2
  Switch1/1 -> Switch2/3
  Size/1(Byte_Count) -> Relational Operator1/1, Relational Operator/1
  Type/1 -> Size/1(Type)
  Data Type Conversion7/1 -> Mux/7  "6"
  Data Type Conversion6/1 -> Mux/6  "5"
  Data Type Conversion5/1 -> Mux/5  "4"
  Data Type Conversion4/1 -> Mux/4  "3"
  Data Type Conversion3/1 -> Mux/3  "2"
  Data Type Conversion2/1 -> Mux/2  "1"
  Data Type Conversion1/1 -> Mux/1  "0"
  Offset/1 -> [offset]
  Data/1 -> Demux/1
  Demux/1 -> Data Type Conversion/1
  Demux/2 -> Data Type Conversion1/1
  Demux/3 -> Data Type Conversion2/1
  Demux/4 -> Data Type Conversion3/1
  Demux/5 -> Data Type Conversion4/1
  Demux/6 -> Data Type Conversion5/1
  Demux/7 -> Data Type Conversion6/1
  Demux/8 -> Data Type Conversion7/1
  Data Type Conversion/1 -> Terminator/1  "PID"

== system EmE_MBD_Blockset/User-Defined Functions/Snoop/CCP_ETC_SS2/CCP_Parameter_Decode/Decode_Signal6/Signal Decode ==
  Raw32 : Inport
  Type : Inport  Port=2
  Coversion : Inport  Port=3
  Bitwise Operator : simulink/Logic and Bit Operations/Bitwise Operator  logicop=AND  UseBitMask=on  BitMask=bin2dec('00000001')  BitMaskRealWorld=Stored Integer
  FLOAT32 : Subsystem
  Integer_Data : Subsystem
  Switch1 : Switch  Criteria=u2 ~= 0
  Unit_Convert : Subsystem
  Out1 : Outport
  wires:
  Coversion/1 -> Unit_Convert/2(Conversion)
  FLOAT32/1(Raw) -> Switch1/3
  Type/1 -> Integer_Data/1(Type), Bitwise Operator/1
  Raw32/1 -> Integer_Data/2(Raw32), FLOAT32/1(Raw32)
  Bitwise Operator/1 -> Switch1/2
  Switch1/1 -> Out1/1
  Integer_Data/1(Raw) -> Unit_Convert/1(Raw)
  Unit_Convert/1(Scaled) -> Switch1/1

== system EmE_MBD_Blockset/User-Defined Functions/Snoop/CCP_ETC_SS2/CCP_Parameter_Decode/Decode_Signal7/Isolate Data ==
  Offset : Inport
  Data : Inport  Port=2
  Type : Inport  Port=3
  1Byte : Subsystem
  2Bytes : Subsystem
  4Bytes : Subsystem
  Constant1 : Constant
  Constant2 : Constant  Value=2
  Data Type Conversion{,1..7} (8 alike) : DataTypeConversion  OutDataTypeStr=uint8
  Demux : Demux  Outputs=8
  Mux : Mux  Inputs=7
  Relational Operator : RelationalOperator  Operator===  OutDataTypeStr=boolean  RndMeth=Nearest
  Relational Operator1 : RelationalOperator  Operator===  OutDataTypeStr=boolean  RndMeth=Nearest
  Size : Subsystem
  Switch1 : Switch  Criteria=u2 ~= 0
  Switch2 : Switch  Criteria=u2 ~= 0
  Terminator : Terminator
  Raw32 : Outport
  wires:
  Data Type Conversion/1 -> Terminator/1  "PID"
  Demux/8 -> Data Type Conversion7/1
  Demux/7 -> Data Type Conversion6/1
  Demux/6 -> Data Type Conversion5/1
  Demux/5 -> Data Type Conversion4/1
  Demux/4 -> Data Type Conversion3/1
  Demux/3 -> Data Type Conversion2/1
  Demux/2 -> Data Type Conversion1/1
  Demux/1 -> Data Type Conversion/1
  Data/1 -> Demux/1
  Offset/1 -> [offset]
  Data Type Conversion1/1 -> Mux/1  "0"
  Data Type Conversion2/1 -> Mux/2  "1"
  Data Type Conversion3/1 -> Mux/3  "2"
  Data Type Conversion4/1 -> Mux/4  "3"
  Data Type Conversion5/1 -> Mux/5  "4"
  Data Type Conversion6/1 -> Mux/6  "5"
  Data Type Conversion7/1 -> Mux/7  "6"
  Type/1 -> Size/1(Type)
  Size/1(Byte_Count) -> Relational Operator/1, Relational Operator1/1
  Switch1/1 -> Switch2/3
  Constant1/1 -> Relational Operator/2
  Constant2/1 -> Relational Operator1/2
  Relational Operator/1 -> Switch2/2
  Relational Operator1/1 -> Switch1/2
  1Byte/1(Y) -> Switch2/1
  [offset] -> 1Byte/2(Idx)
  [data] -> 1Byte/1(U)
  2Bytes/1(Y) -> Switch1/1
  Mux/1 -> 2Bytes/1(U), [data], 4Bytes/1(U)
  [offset] -> 2Bytes/2(Idx1)
  [offset] -> 4Bytes/2(Idx)
  Switch2/1 -> Raw32/1
  4Bytes/1(Y) -> Switch1/3

== system EmE_MBD_Blockset/User-Defined Functions/Snoop/CCP_ETC_SS2/CCP_Parameter_Decode/Decode_Signal7/Signal Decode ==
  Raw32 : Inport
  Type : Inport  Port=2
  Coversion : Inport  Port=3
  Bitwise Operator : simulink/Logic and Bit Operations/Bitwise Operator  logicop=AND  UseBitMask=on  BitMask=bin2dec('00000001')  BitMaskRealWorld=Stored Integer
  FLOAT32 : Subsystem
  Integer_Data : Subsystem
  Switch1 : Switch  Criteria=u2 ~= 0
  Unit_Convert : Subsystem
  Out1 : Outport
  wires:
  Unit_Convert/1(Scaled) -> Switch1/1
  Integer_Data/1(Raw) -> Unit_Convert/1(Raw)
  Switch1/1 -> Out1/1
  Bitwise Operator/1 -> Switch1/2
  Raw32/1 -> FLOAT32/1(Raw32), Integer_Data/2(Raw32)
  Type/1 -> Bitwise Operator/1, Integer_Data/1(Type)
  FLOAT32/1(Raw) -> Switch1/3
  Coversion/1 -> Unit_Convert/2(Conversion)

== system EmE_MBD_Blockset/User-Defined Functions/Snoop/CCP_ETC_SS2/CCP_Parameter_Decode/Decode_Signal8/Isolate Data ==
  Offset : Inport
  Data : Inport  Port=2
  Type : Inport  Port=3
  1Byte : Subsystem
  2Bytes : Subsystem
  4Bytes : Subsystem
  Constant1 : Constant
  Constant2 : Constant  Value=2
  Data Type Conversion{,1..7} (8 alike) : DataTypeConversion  OutDataTypeStr=uint8
  Demux : Demux  Outputs=8
  Mux : Mux  Inputs=7
  Relational Operator : RelationalOperator  Operator===  OutDataTypeStr=boolean  RndMeth=Nearest
  Relational Operator1 : RelationalOperator  Operator===  OutDataTypeStr=boolean  RndMeth=Nearest
  Size : Subsystem
  Switch1 : Switch  Criteria=u2 ~= 0
  Switch2 : Switch  Criteria=u2 ~= 0
  Terminator : Terminator
  Raw32 : Outport
  wires:
  4Bytes/1(Y) -> Switch1/3
  Switch2/1 -> Raw32/1
  [offset] -> 4Bytes/2(Idx)
  [offset] -> 2Bytes/2(Idx1)
  Mux/1 -> 4Bytes/1(U), [data], 2Bytes/1(U)
  2Bytes/1(Y) -> Switch1/1
  [data] -> 1Byte/1(U)
  [offset] -> 1Byte/2(Idx)
  1Byte/1(Y) -> Switch2/1
  Relational Operator1/1 -> Switch1/2
  Relational Operator/1 -> Switch2/2
  Constant2/1 -> Relational Operator1/2
  Constant1/1 -> Relational Operator/2
  Switch1/1 -> Switch2/3
  Size/1(Byte_Count) -> Relational Operator1/1, Relational Operator/1
  Type/1 -> Size/1(Type)
  Data Type Conversion7/1 -> Mux/7  "6"
  Data Type Conversion6/1 -> Mux/6  "5"
  Data Type Conversion5/1 -> Mux/5  "4"
  Data Type Conversion4/1 -> Mux/4  "3"
  Data Type Conversion3/1 -> Mux/3  "2"
  Data Type Conversion2/1 -> Mux/2  "1"
  Data Type Conversion1/1 -> Mux/1  "0"
  Offset/1 -> [offset]
  Data/1 -> Demux/1
  Demux/1 -> Data Type Conversion/1
  Demux/2 -> Data Type Conversion1/1
  Demux/3 -> Data Type Conversion2/1
  Demux/4 -> Data Type Conversion3/1
  Demux/5 -> Data Type Conversion4/1
  Demux/6 -> Data Type Conversion5/1
  Demux/7 -> Data Type Conversion6/1
  Demux/8 -> Data Type Conversion7/1
  Data Type Conversion/1 -> Terminator/1  "PID"

== system EmE_MBD_Blockset/User-Defined Functions/Snoop/CCP_ETC_SS2/CCP_Parameter_Decode/Decode_Signal8/Signal Decode ==
  Raw32 : Inport
  Type : Inport  Port=2
  Coversion : Inport  Port=3
  Bitwise Operator : simulink/Logic and Bit Operations/Bitwise Operator  logicop=AND  UseBitMask=on  BitMask=bin2dec('00000001')  BitMaskRealWorld=Stored Integer
  FLOAT32 : Subsystem
  Integer_Data : Subsystem
  Switch1 : Switch  Criteria=u2 ~= 0
  Unit_Convert : Subsystem
  Out1 : Outport
  wires:
  Coversion/1 -> Unit_Convert/2(Conversion)
  FLOAT32/1(Raw) -> Switch1/3
  Type/1 -> Integer_Data/1(Type), Bitwise Operator/1
  Raw32/1 -> Integer_Data/2(Raw32), FLOAT32/1(Raw32)
  Bitwise Operator/1 -> Switch1/2
  Switch1/1 -> Out1/1
  Integer_Data/1(Raw) -> Unit_Convert/1(Raw)
  Unit_Convert/1(Scaled) -> Switch1/1

== system EmE_MBD_Blockset/User-Defined Functions/Snoop/CCP_ETC_SS2/CCP_Parameter_Decode/Decode_Signal9/Isolate Data ==
  Offset : Inport
  Data : Inport  Port=2
  Type : Inport  Port=3
  1Byte : Subsystem
  2Bytes : Subsystem
  4Bytes : Subsystem
  Constant1 : Constant
  Constant2 : Constant  Value=2
  Data Type Conversion{,1..7} (8 alike) : DataTypeConversion  OutDataTypeStr=uint8
  Demux : Demux  Outputs=8
  Mux : Mux  Inputs=7
  Relational Operator : RelationalOperator  Operator===  OutDataTypeStr=boolean  RndMeth=Nearest
  Relational Operator1 : RelationalOperator  Operator===  OutDataTypeStr=boolean  RndMeth=Nearest
  Size : Subsystem
  Switch1 : Switch  Criteria=u2 ~= 0
  Switch2 : Switch  Criteria=u2 ~= 0
  Terminator : Terminator
  Raw32 : Outport
  wires:
  Data Type Conversion/1 -> Terminator/1  "PID"
  Demux/8 -> Data Type Conversion7/1
  Demux/7 -> Data Type Conversion6/1
  Demux/6 -> Data Type Conversion5/1
  Demux/5 -> Data Type Conversion4/1
  Demux/4 -> Data Type Conversion3/1
  Demux/3 -> Data Type Conversion2/1
  Demux/2 -> Data Type Conversion1/1
  Demux/1 -> Data Type Conversion/1
  Data/1 -> Demux/1
  Offset/1 -> [offset]
  Data Type Conversion1/1 -> Mux/1  "0"
  Data Type Conversion2/1 -> Mux/2  "1"
  Data Type Conversion3/1 -> Mux/3  "2"
  Data Type Conversion4/1 -> Mux/4  "3"
  Data Type Conversion5/1 -> Mux/5  "4"
  Data Type Conversion6/1 -> Mux/6  "5"
  Data Type Conversion7/1 -> Mux/7  "6"
  Type/1 -> Size/1(Type)
  Size/1(Byte_Count) -> Relational Operator/1, Relational Operator1/1
  Switch1/1 -> Switch2/3
  Constant1/1 -> Relational Operator/2
  Constant2/1 -> Relational Operator1/2
  Relational Operator/1 -> Switch2/2
  Relational Operator1/1 -> Switch1/2
  1Byte/1(Y) -> Switch2/1
  [offset] -> 1Byte/2(Idx)
  [data] -> 1Byte/1(U)
  2Bytes/1(Y) -> Switch1/1
  Mux/1 -> 2Bytes/1(U), [data], 4Bytes/1(U)
  [offset] -> 2Bytes/2(Idx1)
  [offset] -> 4Bytes/2(Idx)
  Switch2/1 -> Raw32/1
  4Bytes/1(Y) -> Switch1/3

== system EmE_MBD_Blockset/User-Defined Functions/Snoop/CCP_ETC_SS2/CCP_Parameter_Decode/Decode_Signal9/Signal Decode ==
  Raw32 : Inport
  Type : Inport  Port=2
  Coversion : Inport  Port=3
  Bitwise Operator : simulink/Logic and Bit Operations/Bitwise Operator  logicop=AND  UseBitMask=on  BitMask=bin2dec('00000001')  BitMaskRealWorld=Stored Integer
  FLOAT32 : Subsystem
  Integer_Data : Subsystem
  Switch1 : Switch  Criteria=u2 ~= 0
  Unit_Convert : Subsystem
  Out1 : Outport
  wires:
  Unit_Convert/1(Scaled) -> Switch1/1
  Integer_Data/1(Raw) -> Unit_Convert/1(Raw)
  Switch1/1 -> Out1/1
  Bitwise Operator/1 -> Switch1/2
  Raw32/1 -> FLOAT32/1(Raw32), Integer_Data/2(Raw32)
  Type/1 -> Bitwise Operator/1, Integer_Data/1(Type)
  FLOAT32/1(Raw) -> Switch1/3
  Coversion/1 -> Unit_Convert/2(Conversion)

== system EmE_MBD_Blockset/User-Defined Functions/Snoop/CCP_ETC_SS2/CCP_Parameter_Decode/Decode_Signal1/Isolate Data/1Byte ==
  U : Inport
  Idx : Inport  Port=2
  1Byte : Selector  IndexMode=Zero-based  InputPortWidth=7  IndexOptions=Starting index (port)  Indices=1  OutputSizes=1
  Data Type Conversion : DataTypeConversion  OutDataTypeStr=uint32
  Y : Outport
  wires:
  U/1 -> 1Byte/1
  1Byte/1 -> Data Type Conversion/1
  Idx/1 -> 1Byte/2
  Data Type Conversion/1 -> Y/1

== system EmE_MBD_Blockset/User-Defined Functions/Snoop/CCP_ETC_SS2/CCP_Parameter_Decode/Decode_Signal1/Isolate Data/2Bytes ==
  U : Inport
  Idx1 : Inport  Port=2
  2Byte : Selector  IndexMode=Zero-based  InputPortWidth=7  IndexOptions=Starting index (port)  Indices=1  OutputSizes=2
  Add : Sum
  Constant : Constant  Value=5  OutDataTypeStr=uint8
  Data Type Conversion : DataTypeConversion  OutDataTypeStr=uint32
  Data Type Conversion1 : DataTypeConversion  OutDataTypeStr=uint32
  Demux : Demux  Outputs=2
  Relational Operator : RelationalOperator  Operator=<  OutDataTypeStr=boolean  RndMeth=Nearest
  Shift Arithmetic : ArithShift
  Switch1 : Switch  Criteria=u2 ~= 0
  Y : Outport
  wires:
  Constant/1 -> Relational Operator/1, Switch1/1
  Data Type Conversion/1 -> Y/1
  U/1 -> 2Byte/1
  Demux/2 -> Add/2
  Demux/1 -> Shift Arithmetic/1
  Shift Arithmetic/1 -> Add/1
  Add/1 -> Data Type Conversion/1
  Data Type Conversion1/1 -> Demux/1
  2Byte/1 -> Data Type Conversion1/1
  Relational Operator/1 -> Switch1/2
  Idx1/1 -> Relational Operator/2, Switch1/3
  Switch1/1 -> 2Byte/2

== system EmE_MBD_Blockset/User-Defined Functions/Snoop/CCP_ETC_SS2/CCP_Parameter_Decode/Decode_Signal1/Isolate Data/4Bytes ==
  U : Inport
  Idx : Inport  Port=2
  4Byte : Selector  IndexMode=Zero-based  InputPortWidth=7  IndexOptions=Starting index (port)  Indices=1  OutputSizes=4
  Add : Sum  Inputs=++++
  Constant1 : Constant  Value=3  OutDataTypeStr=uint8
  Data Type Conversion1 : DataTypeConversion  OutDataTypeStr=uint32
  Data Type Conversion2 : DataTypeConversion  OutDataTypeStr=uint32
  Demux : Demux
  Relational Operator1 : RelationalOperator  Operator=<  OutDataTypeStr=boolean  RndMeth=Nearest
  Shift Arithmetic : ArithShift
  Shift Arithmetic1 : ArithShift
  Shift Arithmetic2 : ArithShift
  Switch2 : Switch  Criteria=u2 ~= 0
  Y : Outport
  wires:
  Constant1/1 -> Relational Operator1/1, Switch2/1
  Relational Operator1/1 -> Switch2/2
  Idx/1 -> Relational Operator1/2, Switch2/3
  U/1 -> 4Byte/1
  4Byte/1 -> Data Type Conversion2/1
  Data Type Conversion1/1 -> Y/1
  Demux/2 -> Shift Arithmetic1/1
  Demux/1 -> Shift Arithmetic/1
  Shift Arithmetic/1 -> Add/1
  Add/1 -> Data Type Conversion1/1
  Shift Arithmetic1/1 -> Add/2
  Demux/4 -> Add/4
  Demux/3 -> Shift Arithmetic2/1
  Shift Arithmetic2/1 -> Add/3
  Data Type Conversion2/1 -> Demux/1
  Switch2/1 -> 4Byte/2

== system EmE_MBD_Blockset/User-Defined Functions/Snoop/CCP_ETC_SS2/CCP_Parameter_Decode/Decode_Signal1/Isolate Data/Size ==
  Type : Inport
  Bitwise Operator : simulink/Logic and Bit Operations/Bitwise Operator  logicop=AND  UseBitMask=on  BitMask=bin2dec('00000001')  BitMaskRealWorld=Stored Integer
  Bitwise Operator1 : simulink/Logic and Bit Operations/Bitwise Operator  logicop=AND  UseBitMask=on  BitMask=bin2dec('00000010')  BitMaskRealWorld=Stored Integer
  Bitwise Operator2 : simulink/Logic and Bit Operations/Bitwise Operator  logicop=AND  UseBitMask=on  BitMask=bin2dec('00000100')  BitMaskRealWorld=Stored Integer
  Constant2 : Constant  Value=2
  Constant3 : Constant
  Constant4 : Constant  Value=4
  Logical Operator : Logic  Operator=OR  AllPortsSameDT=off  OutDataTypeStr=boolean
  Logical Operator1 : Logic  Operator=NOT  AllPortsSameDT=off  OutDataTypeStr=boolean
  Switch1 : Switch  Criteria=u2 ~= 0
  Switch2 : Switch  Criteria=u2 ~= 0
  Byte_Count : Outport
  wires:
  Logical Operator/1 -> Switch2/2
  Type/1 -> Bitwise Operator2/1, Bitwise Operator1/1, Bitwise Operator/1
  Bitwise Operator/1 -> Logical Operator1/1
  Switch1/1 -> Switch2/3
  Bitwise Operator2/1 -> Logical Operator/2
  Logical Operator1/1 -> Logical Operator/1
  Bitwise Operator1/1 -> Switch1/2
  Constant2/1 -> Switch1/1
  Constant3/1 -> Switch1/3
  Switch2/1 -> Byte_Count/1
  Constant4/1 -> Switch2/1

== system EmE_MBD_Blockset/User-Defined Functions/Snoop/CCP_ETC_SS2/CCP_Parameter_Decode/Decode_Signal1/Signal Decode/FLOAT32 ==
  note: (-1)^s × c × b^q
  note: S        Q         C
      | 31    30-23    22-0
  Raw32 : Inport
  Add8 : Sum
  Add9 : Sum  Inputs=-+
  Bitwise Operator : simulink/Logic and Bit Operations/Bitwise Operator  logicop=AND  UseBitMask=on  BitMask=bin2dec('10000000000000000000000000000000')  BitMaskRealWorld=Stored Integer
  Bitwise Operator1 : simulink/Logic and Bit Operations/Bitwise Operator  logicop=AND  UseBitMask=on  BitMask=bin2dec('01111111100000000000000000000000')  BitMaskRealWorld=Stored Integer
  Bitwise Operator2 : simulink/Logic and Bit Operations/Bitwise Operator  logicop=AND  UseBitMask=on  BitMask=bin2dec('00000000011111111111111111111111')  BitMaskRealWorld=Stored Integer
  Constant : Constant  Value=10
  Constant5 : Constant  OutDataTypeStr=double
  Constant6 : Constant  Value=2  OutDataTypeStr=double
  Constant7 : Constant  Value=127  OutDataTypeStr=double
  Data Type Conversion{1..8} (8 alike) : DataTypeConversion  OutDataTypeStr=double
  Math Function1 : Math  Operator=pow  SaturateOnIntegerOverflow=on
  Product1 : Product  RndMeth=Zero
  Shift Arithmetic6 : ArithShift
  Shift Arithmetic7 : ArithShift
  Shift Arithmetic8 : ArithShift
  Terminator3 : Terminator
  sign1 : Terminator
  Raw : Outport
  wires:
  Data Type Conversion8/1 -> Product1/1
  Data Type Conversion7/1 -> Product1/2
  Data Type Conversion6/1 -> Add8/1
  Data Type Conversion5/1 -> Add9/1
  Data Type Conversion3/1 -> Shift Arithmetic8/1
  Data Type Conversion1/1 -> Raw/1
  Product1/1 -> Data Type Conversion1/1
  Add8/1 -> Data Type Conversion7/1
  Constant7/1 -> Data Type Conversion5/1
  Data Type Conversion4/1 -> Add9/2
  Math Function1/1 -> Data Type Conversion8/1
  Constant6/1 -> Math Function1/1
  Add9/1 -> Math Function1/2
  Shift Arithmetic7/1 -> Data Type Conversion4/1
  Data Type Conversion2/1 -> Add8/2
  Constant5/1 -> Data Type Conversion6/1
  Shift Arithmetic8/1 -> Data Type Conversion2/1
  Shift Arithmetic6/1 -> sign1/1
  Bitwise Operator/1 -> Shift Arithmetic6/1  "s"
  Bitwise Operator1/1 -> Shift Arithmetic7/1  "q"
  Bitwise Operator2/1 -> Data Type Conversion3/1  "c"
  Raw32/1 -> Bitwise Operator/1, Bitwise Operator1/1, Bitwise Operator2/1
  Constant/1 -> Terminator3/1  "b"
